simulink model "Test_filter"  (R2020b)
settings: Solver=VariableStepAuto  StartTime=0.0  StopTime=10.0  RelTol=1e-3
libraries: dspfdesign x1, dspstat3 x1
settings Model: Creator=alessandro  LastModifiedBy=alessandro

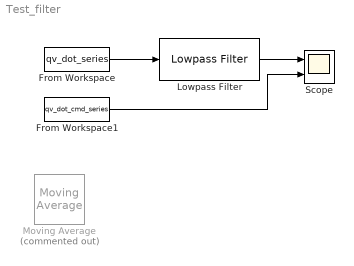
== system Test_filter ==
  From Workspace : FromWorkspace  VariableName=qv_dot_series  OutDataTypeStr=double  SampleTime=0.003
  From Workspace1 : FromWorkspace  VariableName=qv_dot_cmd_series  OutDataTypeStr=double  SampleTime=0.003
  Lowpass Filter : dspfdesign/Lowpass Filter  FilterType=IIR  DesignForMinimumOrder=on  FilterOrder=50  PassbandFrequency=2  StopbandFrequency=5  PassbandRipple=0.1  StopbandAttenuation=40  InheritSampleRate=off  SampleRate=333  SimulateUsing=Interpreted execution  roundingMode=Floor  coeffsDataTypeStr=fixdt(1,16)
  Moving Average : dspstat3/Moving Average  Commented=on  Method=Sliding window  ForgettingFactorPort=off  SpecifyWindowLength=on  WindowLength=10  ForgettingFactor=0.9  SimulateUsing=Code generation
  Scope : Scope  NumInputPorts=2
  wires:
  From Workspace/1 -> Lowpass Filter/1
  Lowpass Filter/1 -> Scope/1
  From Workspace1/1 -> Scope/2
